simulink model "luenberger_observer"  (R2023b)
settings: Solver=FixedStepDiscrete  StartTime=0.0  StopTime=10.0  FixedStep=0.0001  RelTol=1e-3
values from neighbouring files (symbols this model uses):
  B = 0.01    [luenberger_observer_parm.m]
  g1 = 2*wn    (= 2000)    [luenberger_observer_parm.m]
  g2 = -J*wn*wn    (= -100)    [luenberger_observer_parm.m]
  J = 0.0001    [luenberger_observer_parm.m]
  Te = 1    [luenberger_observer_parm.m]
undefined symbols (not defined in the file or in its folder): DiscIntNeverNeededParam
settings Model: Creator=ZJX  LastModifiedBy=ZJX
settings OptimizationCC: BlockReduction=off  DefaultParameterBehavior=Inlined  EnhancedBackFolding=on  PassReuseOutputArgsAs=Individual arguments  ZeroExternalMemoryAtStartup=off  ZeroInternalMemoryAtStartup=off  OptimizeBlockOrder=speed  DifferentSizesBufferReuse=on  OptimizationCustomize=off  EfficientTunableParamExpr=on
settings DebuggingCC: ParameterTunabilityLossMsg=error
settings SFSimCC: MATLABDynamicMemAlloc=off
settings RTWCC: Description=Embedded Coder  SystemTargetFile=ert.tlc  TemplateMakefile=ert_default_tmf
settings CodeAppCC: ForceParamTrailComments=on  IgnoreCustomStorageClasses=off  OperatorAnnotations=on  SimulinkDataObjDesc=on  SFDataObjDesc=on  InsertBlockDesc=on
settings ERTTargetCC: TargetLangStandard=C99 (ISO)  GenerateSampleERTMain=on  InlinedParameterPlacement=NonHierarchical  ERTCustomFileTemplate=example_file_process.tlc

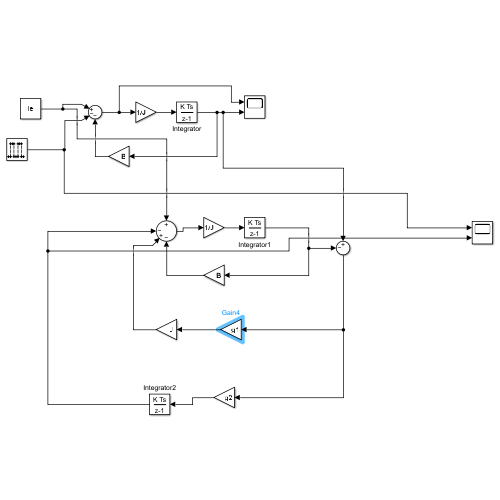
[thumbnail: Simulink's stored preview of the top-level diagram]
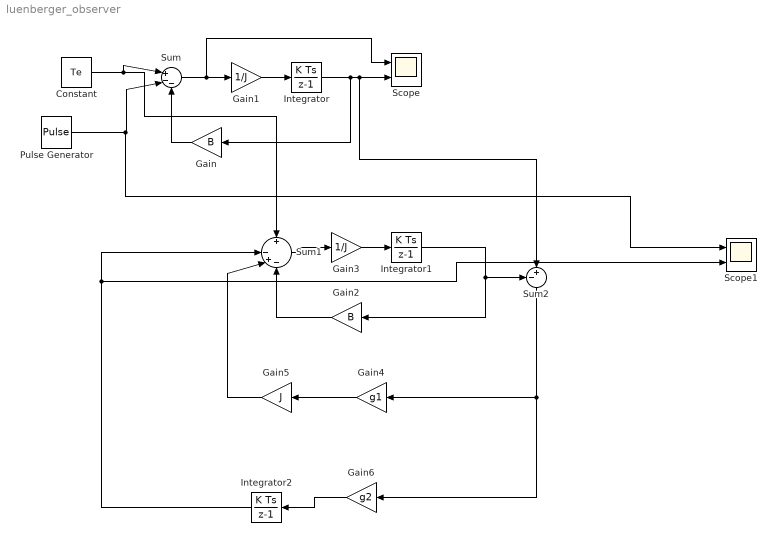
== system luenberger_observer ==
  Constant : Constant  Value=Te
  Gain : Gain  Gain=B
  Gain1 : Gain  Gain=1/J
  Gain2 : Gain  Gain=B
  Gain3 : Gain  Gain=1/J
  Gain4 : Gain  Gain=g1
  Gain5 : Gain  Gain=J
  Gain6 : Gain  Gain=g2
  Integrator : DiscreteIntegrator  SampleTime=0.0001  ICPrevOutput=DiscIntNeverNeededParam  ICPrevScaledInput=DiscIntNeverNeededParam  mask(DiscretizedDiscreteIntegrator){}
      mask init:
      | %zoh
  Integrator1 : DiscreteIntegrator  SampleTime=0.0001  ICPrevOutput=DiscIntNeverNeededParam  ICPrevScaledInput=DiscIntNeverNeededParam  mask(DiscretizedDiscreteIntegrator){}
      mask init:
      | %zoh
  Integrator2 : DiscreteIntegrator  SampleTime=0.0001  ICPrevOutput=DiscIntNeverNeededParam  ICPrevScaledInput=DiscIntNeverNeededParam  mask(DiscretizedDiscreteIntegrator){}
      mask init:
      | %zoh
  Pulse Generator : DiscretePulseGenerator  Amplitude=0.5  Period=10000  PulseWidth=5000  SampleTime=0.000100000000000000005
  Scope : Scope  NumInputPorts=2
  Scope1 : Scope  NumInputPorts=2
  Sum : Sum  Inputs=|+--
  Sum1 : Sum  Inputs=+|-+-
  Sum2 : Sum  Inputs=-+|
  wires:
  Pulse Generator/1 -> Scope1/1, Sum/2
  Gain/1 -> Sum/3
  Sum/1 -> Scope/1, Gain1/1
  Gain1/1 -> Integrator/1
  Constant/1 -> Sum1/1, Sum/1
  Integrator/1 -> Sum2/2, Scope/2, Gain/1
  Integrator2/1 -> Scope1/2, Sum1/2
  Gain4/1 -> Gain5/1
  Gain3/1 -> Integrator1/1
  Gain5/1 -> Sum1/3
  Gain2/1 -> Sum1/4
  Gain6/1 -> Integrator2/1
  Sum2/1 -> Gain6/1, Gain4/1
  Integrator1/1 -> Sum2/1, Gain2/1
  Sum1/1 -> Gain3/1
